simulink model "Lewitacja_LQI"  (R2015a)
settings: Solver=ode5  SolverMode=SingleTasking  StartTime=0.0  StopTime=inf  FixedStep=0.001  RelTol=1e-3  AbsTol=1e-6
PostLoadFcn:
  | load ML_Sensor
values from neighbouring files (symbols this model uses):
  g = model.g    [Levitation.m]
  ki = 2.8964    [Levitation.m]
  m = model.m    [Levitation.m]
  Par_Fem = [DLchar.coefs.a -1/DLchar.coefs.b]    [Levitation.m]
  uc = 0    [Levitation.m]
  x0 = 0    [Levitation.m]
undefined symbols (not defined in the file or in its folder): K, VIchar
undefined symbols (not defined in the file): RTDAC4PCIBaseAddress
settings Model: SimulationMode=external  ExtModeEnableFloating=off  ExtModeTrigDuration=40000  ExtModeTrigDirection=either  ExtModeArchiveFileName=exp01.mat  ExtModeArchiveDirName=h:\temp  ExtModeWriteAllDataToWs=on  Creator=Adam Pilat  LastModifiedBy=Student
settings DataIOCC: ExternalInput=[]  InitialState=[]  LimitDataPoints=off  MaxDataPoints=5000  SignalLoggingSaveFormat=ModelDataLogs  SaveOutput=off  SaveTime=off  SignalLoggingName=sigsOut
settings OptimizationCC: BooleanDataType=off  ExpressionDepthLimit=2147483647  InitFltsAndDblsToZero=on
settings DebuggingCC: SaveWithParameterizedLinksMsg=none  UnderspecifiedInitializationDetection=Classic  MergeDetectMultiDrivingBlocksExec=none  SignalResolutionControl=TryResolveAllWithWarning  MultiTaskDSMMsg=warning  MultiTaskCondExecSysMsg=none  IntegerOverflowMsg=none  FcnCallInpInsideContextMsg=UseLocalSettings  StateNameClashWarn=warning  IntegerSaturationMsg=none
settings HardwareCC: ProdBitPerLong=64  ProdBitPerPointer=64  ProdIntDivRoundTo=Zero  ProdEndianess=LittleEndian  ProdWordSize=64  ProdHWDeviceType=Intel->x86-64  TargetBitPerLong=64  TargetBitPerPointer=64  TargetIntDivRoundTo=Zero  TargetEndianess=LittleEndian  TargetWordSize=64  TargetHWDeviceType=Intel->x86-64
settings RTWCC: SystemTargetFile=rtwin.tlc  TemplateMakefile=RTDAC_win.tmf  Description=Real-Time Windows Target
settings RTWinTargetCC: TargetFcnLib=ansi_tfl_tmw.mat  TargetPreCompLibLocation=C:\Program Files\MATLAB\R2015aSP1\toolbox\sldrt\lib\win64  ModelReferenceCompliant=off  CompOptLevelCompliant=off

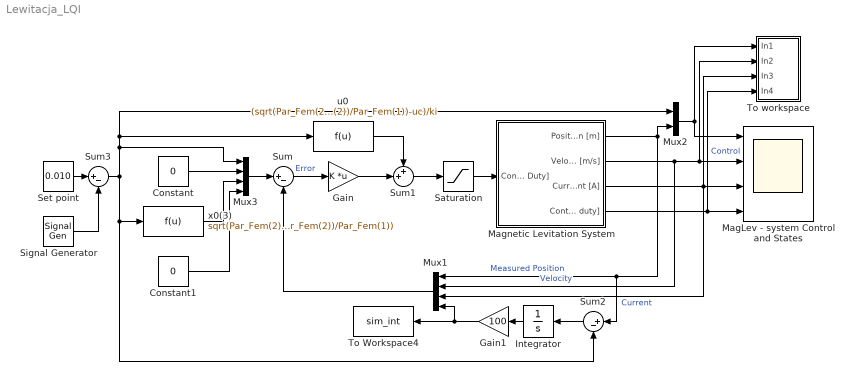
== system Lewitacja_LQI ==
  Constant : Constant  Value=0
  Constant1 : Constant  Value=0
  Gain : Gain  Gain=K  Multiplication=Matrix(K*u)
  Gain1 : Gain  Gain=100
  Integrator : Integrator
  MagLev - system Control and States : Scope  NumInputPorts=4
      settings: TimeRange=10  YMin=0.0055~-0.175~0.6~0  YMax=0.014~0.15~1.4~0.85  SaveName=MLExpData  MaxDataPoints=10000
  Magnetic Levitation System : Subsystem  mask(Magnetic Levitation 1 - System){BA=RTDAC4PCIBaseAddress, T0=0.001}
      mask prompts: BA "Base Address (dec):"; T0 "Sampling period [s]:"
      mask help:
      | MagLev1 - System connection for the real-time operating mode
      | (c) InTeCo 2005
      mask Display: image(imread('MagLev1.tif'))
  Mux1 : Mux
  Mux2 : Mux  Inputs=2
  Mux3 : Mux
  Saturation : Saturate  UpperLimit=1  LowerLimit=0
  Set point : Constant  Value=0.010
  Signal Generator : SignalGenerator  Amplitude=0.002
  Sum : Sum  Inputs=|+-
  Sum1 : Sum  Inputs=++|
  Sum2 : Sum  Inputs=|+-
  Sum3 : Sum  Inputs=|+-
  To Workspace4 : ToWorkspace  VariableName=sim_int  SampleTime=-1
  To workspace : Subsystem
  u0 : Fcn  Expr=(sqrt(Par_Fem(2)*m*g*exp(x0(1)/Par_Fem(2))/Par_Fem(1))-uc)/ki
  x0(3) : Fcn  Expr=sqrt(Par_Fem(2)*m*g*exp(u/Par_Fem(2))/Par_Fem(1))
  wires:
  Magnetic Levitation System/4(Control [PWM duty]) -> To workspace/4(In4), MagLev - system Control and States/4  "Control"
  Mux2/1 -> To workspace/1(In1), MagLev - system Control and States/1
  Magnetic Levitation System/2(Velocity [m/s]) -> Mux1/2, To workspace/2(In2), MagLev - system Control and States/2  "Velocity"
  Magnetic Levitation System/3(Current [A]) -> MagLev - system Control and States/3, Mux1/3, To workspace/3(In3)  "Current"
  Magnetic Levitation System/1(Position [m]) -> Sum2/1, Mux1/1, Mux2/2  "Measured Position"
  Mux1/1 -> Sum/2
  Sum/1 -> Gain/1  "Error"
  Gain/1 -> Sum1/2
  Sum3/1 -> Mux2/1, u0/1, Mux3/1, Sum2/2, x0(3)/1
  u0/1 -> Sum1/1
  Mux3/1 -> Sum/1
  x0(3)/1 -> Mux3/3
  Constant/1 -> Mux3/2
  Constant1/1 -> Mux3/4
  Integrator/1 -> Gain1/1
  Set point/1 -> Sum3/1
  Sum2/1 -> Integrator/1
  Gain1/1 -> Mux1/4, To Workspace4/1
  Saturation/1 -> Magnetic Levitation System/1(Control [PWM Duty])
  Sum1/1 -> Saturation/1
  Signal Generator/1 -> Sum3/2

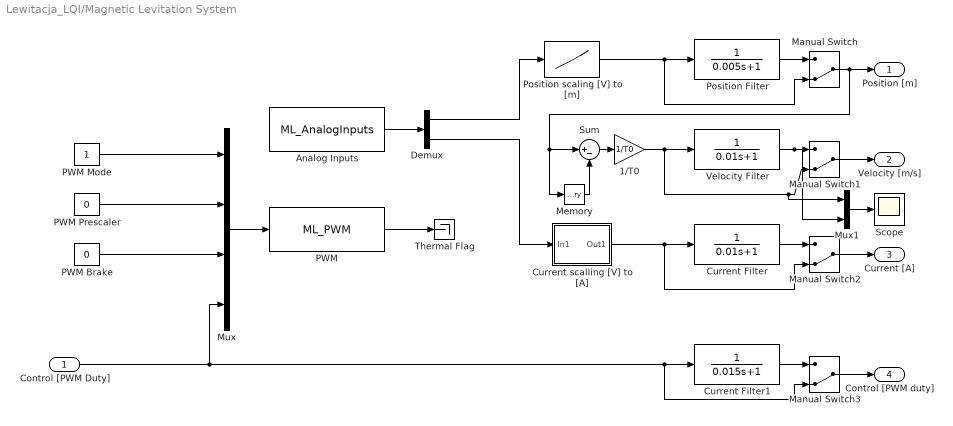
== system Lewitacja_LQI/Magnetic Levitation System ==
  Control [PWM Duty] : Inport
  1/T0 : Gain  Gain=1/T0  SaturateOnIntegerOverflow=on  OutDataTypeStr=Inherit: Same as input  ParamDataTypeStr=Inherit: Same as input
  Analog Inputs : S-Function  FunctionName=ML_AnalogInputs  Parameters=BA, [4 2], [1 1], T0
  Current Filter : TransferFcn  Denominator=[0.01 1]
  Current Filter1 : TransferFcn  Denominator=[0.015 1]
  Current scalling [V] to [A] : Subsystem
      mask Display: plot([0    0.5000    1.0000    1.5000    2.0000    2.5000], [-0.0317    0.4951    1.0302    1.5738    2.1258    2.6863]);
  Demux : Demux  Outputs=2
  Manual Switch{,1..3} (4 alike) : ManualSwitch  CurrentSetting=0
  Memory : Memory
  Mux : Mux
  Mux1 : Mux  Inputs=2
  PWM : S-Function  FunctionName=ML_PWM  Parameters=BA, T0
  PWM Brake : Constant  Value=0
  PWM Mode : Constant
  PWM Prescaler : Constant  Value=0
  Position Filter : TransferFcn  Denominator=[0.005 1]
  Position scaling [V] to [m] : Lookup  InputValues=sensor.V(end:-1:1)  Table=sensor.d(end:-1:1)  SaturateOnIntegerOverflow=on
  Scope : Scope
      settings: YMin=-0.15  YMax=0.125
  Sum : Sum  Inputs=|+-  SaturateOnIntegerOverflow=on  InputSameDT=on  OutDataTypeStr=Inherit: Same as first input
  Thermal Flag : Terminator
  Velocity Filter : TransferFcn  Denominator=[0.01 1]
  Position [m] : Outport
  Velocity [m/s] : Outport  Port=2
  Current [A] : Outport  Port=3
  Control [PWM duty] : Outport  Port=4
  wires:
  Current Filter/1 -> Manual Switch2/1
  Velocity Filter/1 -> Mux1/2, Manual Switch1/1
  Manual Switch/1 -> Position [m]/1, Memory/1, Sum/1
  Position Filter/1 -> Manual Switch/1
  Position scaling [V] to [m]/1 -> Manual Switch/2, Position Filter/1
  Demux/1 -> Position scaling [V] to [m]/1
  Demux/2 -> Current scalling [V] to [A]/1(In1)
  Current scalling [V] to [A]/1(Out1) -> Manual Switch2/2, Current Filter/1
  1/T0/1 -> Mux1/1, Manual Switch1/2, Velocity Filter/1
  Sum/1 -> 1/T0/1
  Memory/1 -> Sum/2
  Analog Inputs/1 -> Demux/1
  Mux/1 -> PWM/1
  PWM Prescaler/1 -> Mux/2
  PWM Mode/1 -> Mux/1
  PWM/1 -> Thermal Flag/1
  Control [PWM Duty]/1 -> Current Filter1/1, Manual Switch3/2, Mux/4
  Manual Switch2/1 -> Current [A]/1
  PWM Brake/1 -> Mux/3
  Manual Switch1/1 -> Velocity [m/s]/1
  Current Filter1/1 -> Manual Switch3/1
  Manual Switch3/1 -> Control [PWM duty]/1
  Mux1/1 -> Scope/1

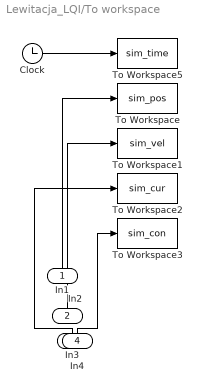
== system Lewitacja_LQI/To workspace ==
  In1 : Inport
  In2 : Inport  Port=2
  In3 : Inport  Port=3
  In4 : Inport  Port=4
  Clock : Clock
  To Workspace : ToWorkspace  VariableName=sim_pos  SampleTime=-1
  To Workspace1 : ToWorkspace  VariableName=sim_vel  SampleTime=-1
  To Workspace2 : ToWorkspace  VariableName=sim_cur  SampleTime=-1
  To Workspace3 : ToWorkspace  VariableName=sim_con  SampleTime=-1
  To Workspace5 : ToWorkspace  VariableName=sim_time  SampleTime=-1
  wires:
  In3/1 -> To Workspace2/1
  Clock/1 -> To Workspace5/1
  In1/1 -> To Workspace/1
  In4/1 -> To Workspace3/1
  In2/1 -> To Workspace1/1

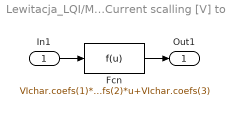
== system Lewitacja_LQI/Magnetic Levitation System/Current scalling [V] to [A] ==
  In1 : Inport
  Fcn : Fcn  Expr=VIchar.coefs(1)*u^2+VIchar.coefs(2)*u+VIchar.coefs(3)
  Out1 : Outport
  wires:
  In1/1 -> Fcn/1
  Fcn/1 -> Out1/1
